simulink model "Simplified_Sim"  (R2018b)
settings: Solver=FixedStepAuto  StartTime=0.0  StopTime=400  RelTol=1e-3  EnableMultiTasking=on
values from neighbouring files (symbols this model uses):
  GPS_time = [129600; 2034]    [sgp4_attitude_test_init.m]
  shifted_epoch = t0    [sgp4_attitude_test_init.m]
undefined symbols (not defined in the file or in its folder): ATMO_ON, clock_lib, DiscIntNeverNeededParam, GG_ON, GPS_time_lib, satelliteDynamics_lib, sgp4, simParams, SP_ON, time_coord_rotation_lib
libraries: aerolibutil x3, gravityGrad_Lib x1, atmoDrag_lib x1, magField_lib x1, solarPressure_lib x1, tle2OE_lib x1, time_Lib x1, attitude_estimation_lib x1, vrlib x1, sgp4_lib_fsw x1, coord_rotation_lib x1, time_conversion_lib x1
settings Model: Creator=devantormey  LastModifiedBy=devantormey
settings OptimizationCC: LifeSpan=inf
settings DebuggingCC: SFUnexpectedBacktrackingDiag=warning  SFNoUnconditionalDefaultTransitionDiag=warning
settings SFSimCC: SimUseLocalCustomCode=off
settings RTWCC: RTWUseLocalCustomCode=off
settings CodeAppCC: StateflowObjectComments=on
settings GRTTargetCC: TargetLangStandard=C89/C90 (ANSI)  GeneratePreprocessorConditionals=Disable all
settings ConfigComp: CovMetricSettings=dw  CovHtmlReporting=on  CovSaveCumulativeToWorkspaceVar=on  CovSaveSingleToWorkspaceVar=on  CovExternalEMLEnable=off

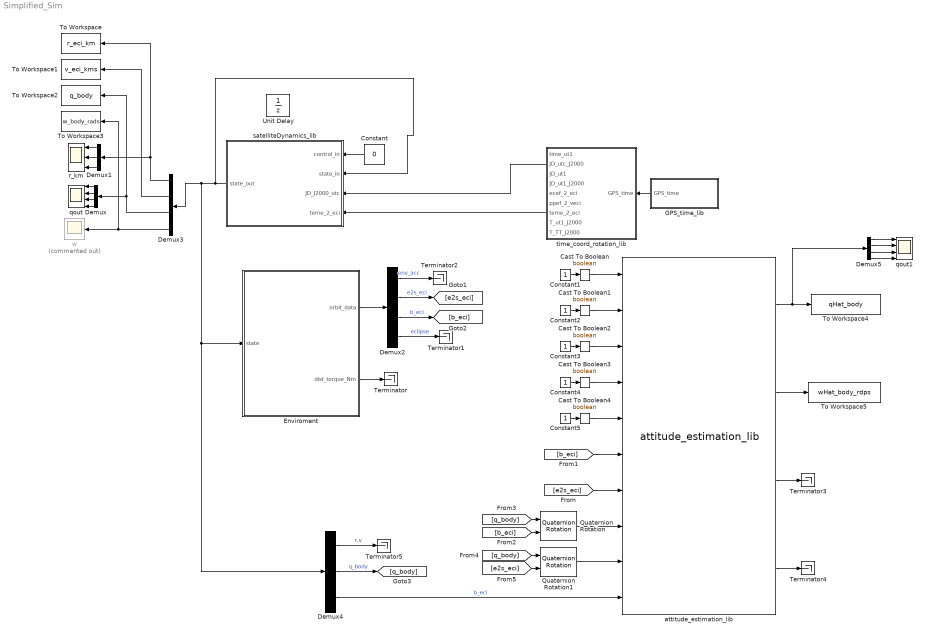
== system Simplified_Sim ==
  Cast To Boolean{,1..4} (5 alike) : DataTypeConversion  OutDataTypeStr=boolean
  Constant : Constant  Value=0
  Constant{1..5} (5 alike) : Constant
  Demux : Demux
  Demux1 : Demux  Outputs=3
  Demux2 : Demux  Outputs=[3 3 3 1]
  Demux3 : Demux  Outputs=[3 3 4 3]
  Demux4 : Demux  Outputs=[6 4 3]
  Demux5 : Demux
  Enviroment : Subsystem
  GPS_time_lib : Subsystem  AncestorBlock=GPS_time_lib/GPS_time_lib
  Quaternion Rotation : aerolibutil/Quaternion Rotation
  Quaternion Rotation1 : aerolibutil/Quaternion Rotation
  Terminator{,1..5} (6 alike) : Terminator
  To Workspace : ToWorkspace  VariableName=r_eci_km  SaveFormat=Timeseries  SampleTime=-1
  To Workspace1 : ToWorkspace  VariableName=v_eci_kms  SaveFormat=Timeseries  SampleTime=-1
  To Workspace2 : ToWorkspace  VariableName=q_body  SaveFormat=Timeseries  SampleTime=-1
  To Workspace3 : ToWorkspace  VariableName=w_body_rads  SaveFormat=Timeseries  SampleTime=-1
  To Workspace4 : ToWorkspace  VariableName=qHat_body  SaveFormat=Timeseries  SampleTime=-1
  To Workspace5 : ToWorkspace  VariableName=wHat_body_rdps  SaveFormat=Timeseries  SampleTime=-1
  Unit Delay : UnitDelay  InitialCondition=[simParams.initialConditions.r0;simParams.initialConditions.v0;simParams.initialConditions.q0;simParams.initialConditions.w0]  SampleTime=-1
  attitude_estimation_lib : attitude_estimation_lib/attitude_estimation_lib  SystemSampleTime=-1
  qout : Scope  NumInputPorts=4
  qout1 : Scope  NumInputPorts=4
  r_km : Scope  NumInputPorts=3
  satelliteDynamics_lib : Subsystem  AncestorBlock=satelliteDynamics_lib/satelliteDynamics_lib
  time_coord_rotation_lib : Subsystem  AncestorBlock=time_coord_rotation_lib/time_coord_rotation_lib
  w : Scope  Commented=on
  wires:
  Demux/1 -> qout/1
  Demux/2 -> qout/2
  Demux/3 -> qout/3
  Demux/4 -> qout/4
  Demux3/3 -> To Workspace2/1, Demux/1
  Demux3/4 -> w/1, To Workspace3/1
  Demux1/3 -> r_km/3
  Demux1/1 -> r_km/1
  Demux1/2 -> r_km/2
  Demux3/1 -> To Workspace/1, Demux1/1
  Demux3/2 -> To Workspace1/1
  Constant/1 -> satelliteDynamics_lib/1(control_in)
  GPS_time_lib/1(GPS_time) -> time_coord_rotation_lib/1(GPS_time)
  time_coord_rotation_lib/2(JD_utc_J2000) -> satelliteDynamics_lib/3(JD_J2000_utc)
  time_coord_rotation_lib/7(teme_2_eci) -> satelliteDynamics_lib/4(teme_2_eci)
  Enviroment/2(dist_torque_Nm) -> Terminator/1
  Enviroment/1(orbit_data) -> Demux2/1
  Demux2/4 -> Terminator1/1  "eclipse"
  Demux2/1 -> Terminator2/1  "env_acc"
  Demux2/2 -> [e2s_eci]  "e2s_eci"
  Demux2/3 -> [b_eci]  "b_eci"
  attitude_estimation_lib/2 -> To Workspace5/1
  attitude_estimation_lib/3 -> Terminator3/1
  Constant1/1 -> Cast To Boolean/1
  Constant2/1 -> Cast To Boolean1/1
  Constant3/1 -> Cast To Boolean2/1
  Constant4/1 -> Cast To Boolean3/1
  Constant5/1 -> Cast To Boolean4/1
  satelliteDynamics_lib/1(state_out) -> satelliteDynamics_lib/2(state_in), Demux4/1, Enviroment/1(state), Demux3/1
  Demux4/1 -> Terminator5/1  "r,v"
  Demux4/2 -> [q_body]  "q_body"
  [b_eci] -> Quaternion Rotation/2
  [q_body] -> Quaternion Rotation/1
  [q_body] -> Quaternion Rotation1/1
  [e2s_eci] -> Quaternion Rotation1/2
  Demux5/1 -> qout1/1
  Demux5/3 -> qout1/3
  Demux5/2 -> qout1/2
  Demux5/4 -> qout1/4
  Cast To Boolean/1 -> attitude_estimation_lib/1
  Cast To Boolean1/1 -> attitude_estimation_lib/2
  Cast To Boolean2/1 -> attitude_estimation_lib/3
  Cast To Boolean3/1 -> attitude_estimation_lib/4
  Cast To Boolean4/1 -> attitude_estimation_lib/5
  [b_eci] -> attitude_estimation_lib/6
  [e2s_eci] -> attitude_estimation_lib/7
  Quaternion Rotation/1 -> attitude_estimation_lib/8
  Quaternion Rotation1/1 -> attitude_estimation_lib/9
  Demux4/3 -> attitude_estimation_lib/10  "b_eci"
  attitude_estimation_lib/4 -> Terminator4/1
  attitude_estimation_lib/1 -> Demux5/1, To Workspace4/1

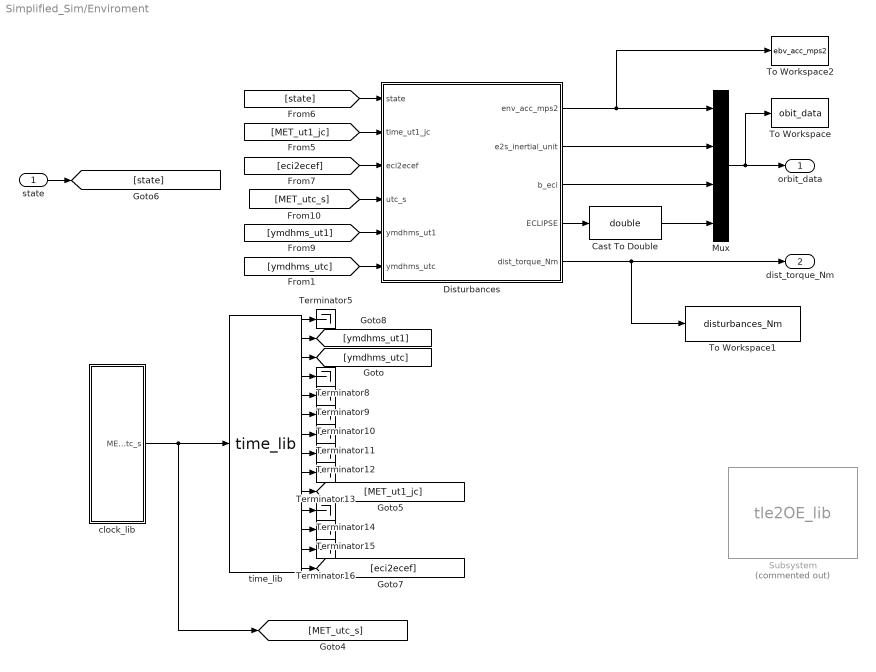
== system Simplified_Sim/Enviroment ==
  state : Inport
  Cast To Double : DataTypeConversion  OutDataTypeStr=double
  Disturbances : Subsystem
  Mux : Mux  Inputs=[3 3 3 1]
  Subsystem : tle2OE_lib/tle2OE_lib  Commented=on  SystemSampleTime=-1
  Terminator{5,8..16} (10 alike) : Terminator
  To Workspace : ToWorkspace  VariableName=obit_data  SaveFormat=Timeseries  SampleTime=-1
  To Workspace1 : ToWorkspace  VariableName=disturbances_Nm  SaveFormat=Timeseries  SampleTime=-1
  To Workspace2 : ToWorkspace  VariableName=ebv_acc_mps2  SaveFormat=Timeseries  SampleTime=-1
  clock_lib : Subsystem  AncestorBlock=clock_lib/clock_lib
  "time_lib " : time_Lib/time_lib    SystemSampleTime=-1
  orbit_data : Outport
  dist_torque_Nm : Outport  Port=2
  wires:
  state/1 -> [state]
  clock_lib/1(MET_utc_s) -> [MET_utc_s], "time_lib "/1
  "time_lib "/10 -> [MET_ut1_jc]
  "time_lib "/14 -> [eci2ecef]
  [eci2ecef] -> Disturbances/3(eci2ecef)
  Disturbances/5(dist_torque_Nm) -> dist_torque_Nm/1, To Workspace1/1
  Disturbances/1(env_acc_mps2) -> To Workspace2/1, Mux/1
  Disturbances/2(e2s_inertial_unit) -> Mux/2
  Mux/1 -> To Workspace/1, orbit_data/1
  [MET_ut1_jc] -> Disturbances/2(time_ut1_jc)
  [state] -> Disturbances/1(state)
  Cast To Double/1 -> Mux/4
  Disturbances/4(ECLIPSE) -> Cast To Double/1
  "time_lib "/1 -> Terminator5/1
  "time_lib "/2 -> [ymdhms_ut1]
  "time_lib "/3 -> [ymdhms_utc]
  "time_lib "/4 -> Terminator8/1
  "time_lib "/5 -> Terminator9/1
  "time_lib "/6 -> Terminator10/1
  "time_lib "/7 -> Terminator11/1
  "time_lib "/8 -> Terminator12/1
  "time_lib "/9 -> Terminator13/1
  "time_lib "/11 -> Terminator14/1
  "time_lib "/12 -> Terminator15/1
  "time_lib "/13 -> Terminator16/1
  [MET_utc_s] -> Disturbances/4(utc_s)
  [ymdhms_ut1] -> Disturbances/5(ymdhms_ut1)
  [ymdhms_utc] -> Disturbances/6(ymdhms_utc)
  Disturbances/3(b_eci) -> Mux/3

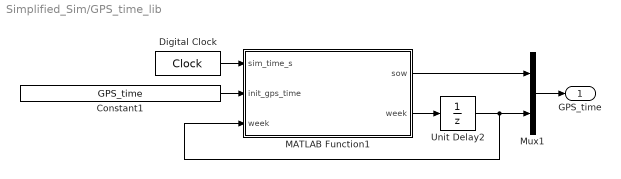
== system Simplified_Sim/GPS_time_lib ==
  Constant1 : Constant  Value=GPS_time  VectorParams1D=off  SampleTime=-1
  Digital Clock : DigitalClock  SampleTime=.1
  MATLAB Function1 : MATLAB Function  TreatAsAtomicUnit=on
  Mux1 : Mux  Inputs=2
  Unit Delay2 : UnitDelay  InitialCondition=GPS_time(2)  SampleTime=-1
  GPS_time : Outport
  wires:
  Mux1/1 -> GPS_time/1
  MATLAB Function1/1(sow) -> Mux1/1
  Unit Delay2/1 -> Mux1/2, MATLAB Function1/3("week ")
  MATLAB Function1/2(week) -> Unit Delay2/1
  Constant1/1 -> MATLAB Function1/2(init_gps_time)
  Digital Clock/1 -> MATLAB Function1/1(sim_time_s)

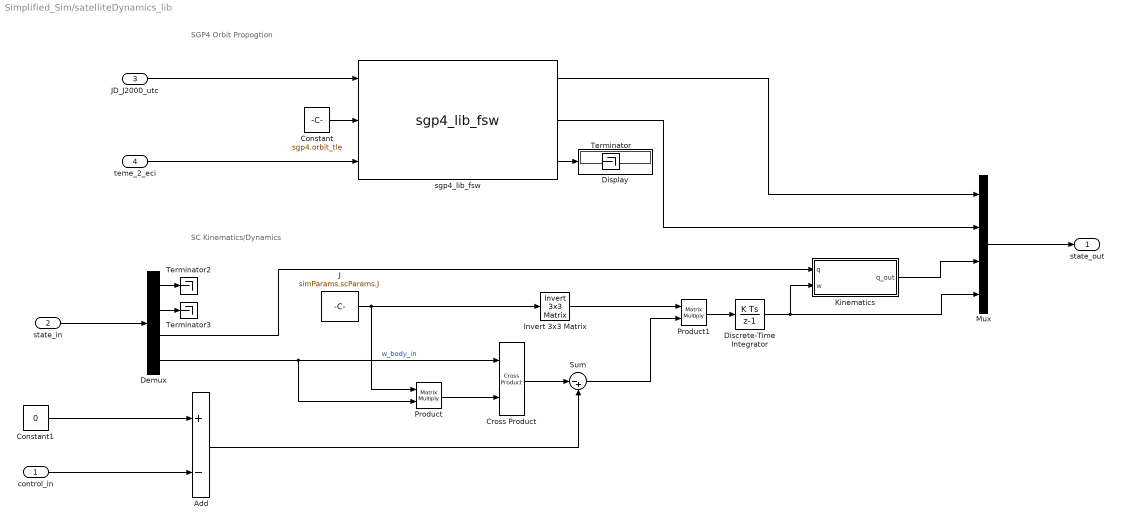
== system Simplified_Sim/satelliteDynamics_lib ==
  note: SC Kinematics/Dynamics
  note: SGP4 Orbit Propogtion
  control_in : Inport
  state_in : Inport  Port=2
  JD_J2000_utc : Inport  Port=3
  teme_2_eci : Inport  Port=4
  Add : Sum  Inputs=+-
  Constant : Constant  Value=sgp4.orbit_tle
  Constant1 : Constant  Value=0
  Cross Product : vrlib/Utilities/Cross Product
      settings: SourceProductBaseCode=VR
  Demux : Demux  Outputs=[3 3 4 3]
  Discrete-Time Integrator : DiscreteIntegrator  InitialCondition=simParams.initialConditions.w0  SampleTime=-1  ICPrevOutput=DiscIntNeverNeededParam  ICPrevScaledInput=DiscIntNeverNeededParam
  Display : Display
  Invert 3x3 Matrix : aerolibutil/Invert  3x3 Matrix
  J : Constant  Value=simParams.scParams.J
  Kinematics : Subsystem
  Mux : Mux  Inputs=[3 3 4 3]
  Product : Product  Multiplication=Matrix(*)
  Product1 : Product  Multiplication=Matrix(*)
  Sum : Sum  Inputs=|-+
  Terminator : Terminator
  Terminator2 : Terminator
  Terminator3 : Terminator
  sgp4_lib_fsw : sgp4_lib_fsw/sgp4_lib_fsw  SystemSampleTime=-1
  state_out : Outport
  wires:
  Demux/2 -> Terminator3/1
  Add/1 -> Sum/2
  control_in/1 -> Add/2
  Constant1/1 -> Add/1
  state_in/1 -> Demux/1
  Mux/1 -> state_out/1
  Demux/1 -> Terminator2/1
  Demux/3 -> Kinematics/1(q)
  Demux/4 -> Product/2, Cross Product/1  "w_body_in"
  Kinematics/1(q_out) -> Mux/3
  Discrete-Time Integrator/1 -> Kinematics/2(w), Mux/4
  Product1/1 -> Discrete-Time Integrator/1
  Invert 3x3 Matrix/1 -> Product1/1
  Sum/1 -> Product1/2
  Cross Product/1 -> Sum/1
  Product/1 -> Cross Product/2
  J/1 -> Invert 3x3 Matrix/1, Product/1
  sgp4_lib_fsw/1 -> Mux/1
  sgp4_lib_fsw/2 -> Mux/2
  sgp4_lib_fsw/3 -> Display/1
  Constant/1 -> sgp4_lib_fsw/2
  teme_2_eci/1 -> sgp4_lib_fsw/3
  JD_J2000_utc/1 -> sgp4_lib_fsw/1

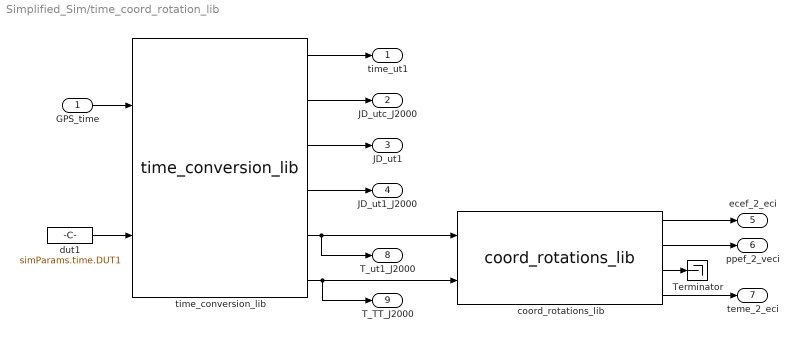
== system Simplified_Sim/time_coord_rotation_lib ==
  GPS_time : Inport
  Terminator : Terminator
  coord_rotations_lib : coord_rotation_lib/coord_rotations_lib  SystemSampleTime=-1
  dut1 : Constant  Value=simParams.time.DUT1
  time_conversion_lib : time_conversion_lib/time_conversion_lib  SystemSampleTime=-1
  time_ut1 : Outport
  JD_utc_J2000 : Outport  Port=2
  JD_ut1 : Outport  Port=3
  JD_ut1_J2000 : Outport  Port=4
  ecef_2_eci : Outport  Port=5
  ppef_2_veci : Outport  Port=6
  teme_2_eci : Outport  Port=7
  T_ut1_J2000 : Outport  Port=8
  T_TT_J2000 : Outport  Port=9
  wires:
  dut1/1 -> time_conversion_lib/2
  time_conversion_lib/5 -> T_ut1_J2000/1, coord_rotations_lib/1
  time_conversion_lib/6 -> T_TT_J2000/1, coord_rotations_lib/2
  time_conversion_lib/1 -> time_ut1/1
  time_conversion_lib/3 -> JD_ut1/1
  time_conversion_lib/4 -> JD_ut1_J2000/1
  coord_rotations_lib/1 -> ecef_2_eci/1
  coord_rotations_lib/2 -> ppef_2_veci/1
  coord_rotations_lib/4 -> teme_2_eci/1
  coord_rotations_lib/3 -> Terminator/1
  time_conversion_lib/2 -> JD_utc_J2000/1
  GPS_time/1 -> time_conversion_lib/1

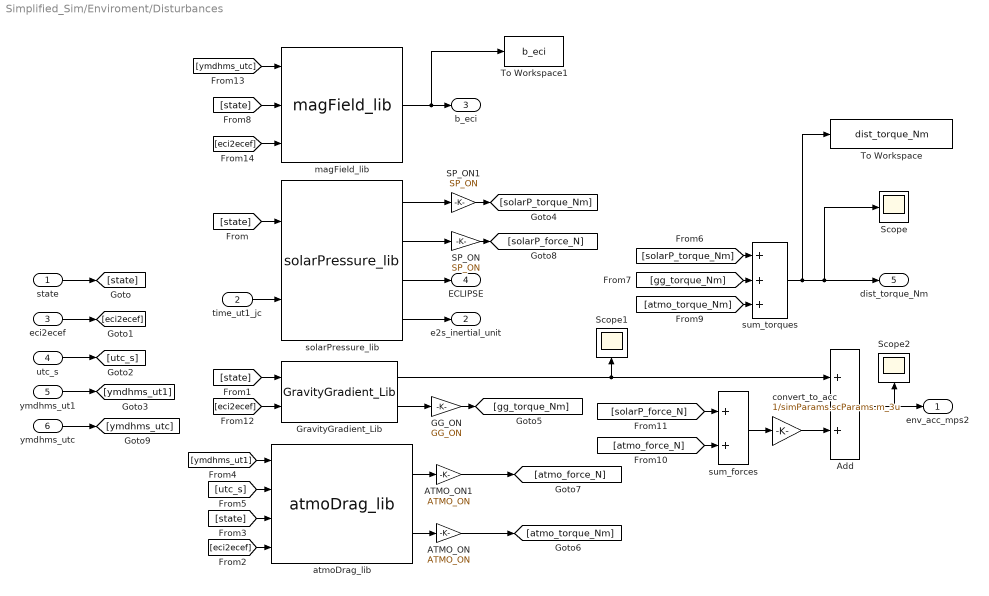
== system Simplified_Sim/Enviroment/Disturbances ==
  state : Inport
  time_ut1_jc : Inport  Port=2
  eci2ecef : Inport  Port=3
  utc_s : Inport  Port=4
  ymdhms_ut1 : Inport  Port=5
  ymdhms_utc : Inport  Port=6
  ATMO_ON : Gain  Gain=ATMO_ON
  ATMO_ON1 : Gain  Gain=ATMO_ON
  Add : Sum
  GG_ON : Gain  Gain=GG_ON
  "GravityGradient_Lib " : gravityGrad_Lib/GravityGradient_Lib   SystemSampleTime=-1
  SP_ON : Gain  Gain=SP_ON
  "SP_ON1 " : Gain  Gain=SP_ON
  Scope : Scope
  Scope1 : Scope
  Scope2 : Scope
  To Workspace : ToWorkspace  VariableName=dist_torque_Nm  SaveFormat=Timeseries  SampleTime=-1
  To Workspace1 : ToWorkspace  VariableName=b_eci  SaveFormat=Timeseries  SampleTime=-1
  atmoDrag_lib : atmoDrag_lib/atmoDrag_lib  SystemSampleTime=-1
  convert_to_acc : Gain  Gain=1/simParams.scParams.m_3u
  magField_lib : magField_lib/magField_lib  SystemSampleTime=-1
      link override Rate Transition2: InitialCondition=0
  solarPressure_lib : solarPressure_lib/solarPressure_lib  SystemSampleTime=-1
  sum_forces : Sum
  sum_torques : Sum  Inputs=+++
  env_acc_mps2 : Outport
  e2s_inertial_unit : Outport  Port=2
  b_eci : Outport  Port=3
  ECLIPSE : Outport  Port=4
  dist_torque_Nm : Outport  Port=5
  wires:
  solarPressure_lib/3 -> ECLIPSE/1
  solarPressure_lib/1 -> "SP_ON1 "/1
  solarPressure_lib/4 -> e2s_inertial_unit/1
  solarPressure_lib/2 -> SP_ON/1
  time_ut1_jc/1 -> solarPressure_lib/2
  sum_forces/1 -> convert_to_acc/1
  Add/1 -> env_acc_mps2/1, Scope2/1
  convert_to_acc/1 -> Add/2
  atmoDrag_lib/2 -> ATMO_ON/1
  atmoDrag_lib/1 -> ATMO_ON1/1
  ATMO_ON/1 -> [atmo_torque_Nm]
  state/1 -> [state]
  [state] -> solarPressure_lib/1
  [state] -> "GravityGradient_Lib "/1
  eci2ecef/1 -> [eci2ecef]
  [eci2ecef] -> atmoDrag_lib/4
  [state] -> atmoDrag_lib/3
  utc_s/1 -> [utc_s]
  ymdhms_ut1/1 -> [ymdhms_ut1]
  [ymdhms_ut1] -> atmoDrag_lib/1
  [utc_s] -> atmoDrag_lib/2
  "SP_ON1 "/1 -> [solarP_torque_Nm]
  [solarP_torque_Nm] -> sum_torques/1
  GG_ON/1 -> [gg_torque_Nm]
  [gg_torque_Nm] -> sum_torques/2
  [eci2ecef] -> "GravityGradient_Lib "/2
  sum_torques/1 -> To Workspace/1, Scope/1, dist_torque_Nm/1
  [atmo_torque_Nm] -> sum_torques/3
  [atmo_force_N] -> sum_forces/2
  [solarP_force_N] -> sum_forces/1
  ATMO_ON1/1 -> [atmo_force_N]
  SP_ON/1 -> [solarP_force_N]
  "GravityGradient_Lib "/1 -> Add/1, Scope1/1
  "GravityGradient_Lib "/2 -> GG_ON/1
  [state] -> magField_lib/2
  ymdhms_utc/1 -> [ymdhms_utc]
  [ymdhms_utc] -> magField_lib/1
  [eci2ecef] -> magField_lib/3
  magField_lib/1 -> To Workspace1/1, b_eci/1

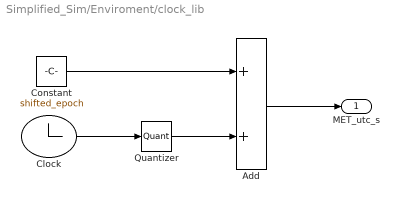
== system Simplified_Sim/Enviroment/clock_lib ==
  Add : Sum
  Clock : Clock
  Constant : Constant  Value=shifted_epoch
  Quantizer : Quantizer  QuantizationInterval=simParams.time.res
  MET_utc_s : Outport
  wires:
  Add/1 -> MET_utc_s/1
  Quantizer/1 -> Add/2
  Constant/1 -> Add/1
  Clock/1 -> Quantizer/1

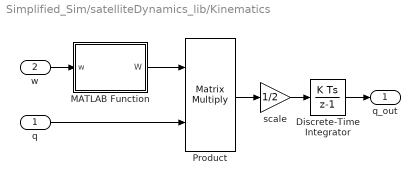
== system Simplified_Sim/satelliteDynamics_lib/Kinematics ==
  q : Inport
  w : Inport  Port=2
  Discrete-Time Integrator : DiscreteIntegrator  InitialCondition=simParams.initialConditions.q0  SampleTime=-1  ICPrevOutput=DiscIntNeverNeededParam  ICPrevScaledInput=DiscIntNeverNeededParam
  MATLAB Function : MATLAB Function  TreatAsAtomicUnit=on
  Product : Product  Multiplication=Matrix(*)
  scale : Gain  Gain=1/2
  q_out : Outport
  wires:
  Discrete-Time Integrator/1 -> q_out/1
  scale/1 -> Discrete-Time Integrator/1
  Product/1 -> scale/1
  q/1 -> Product/2
  MATLAB Function/1(W) -> Product/1
  w/1 -> MATLAB Function/1(w)

== matlab function Simplified_Sim/satelliteDynamics_lib/Kinematics/MATLAB Function ==
  data: w input; W output
function W = fcn(w)
%#codegen

W = [0, -w(1),-w(2),-w(3); w(1), 0,w(3), -w(2); w(2), -w(3), 0, w(1); w(3), w(2), -w(1), 0 ];

end

== matlab function Simplified_Sim/GPS_time_lib/MATLAB Function1 ==
  data: sim_time_s input; sow output; init_gps_time input; week input; week output
function [sow, week] = gps_clock(sim_time_s, init_gps_time, week)
% ----------------------------------------------------------------------- %
% UW HuskySat-1, ADCS Subsystem
%
% GPS clock for the SIM.
% ----------------------------------------------------------------------- %

% Constants
sec_in_week = 604800;


init_sow    = init_gps_time(1);
sow         = mod(init_sow + sim_time_s, sec_in_week);

% Handle roll overs
if sow == sec_in_week
    week = week + 1;
end

end
